simulink model "slexHARFixedPointExample"  (R2023a)
settings: Solver=FixedStepAuto  StartTime=0.0  StopTime=numSteps  FixedStep=1  RelTol=1e-3
PreLoadFcn:
  | % Pre-processing parameters
  | s = [1.0000   -1.0000         0    1.0000   -0.9004         0
  |     1.0000   -1.9996    1.0000    1.0000   -1.9203    0.9254
  |     1.0000   -1.9990    1.0000    1.0000   -1.9762    0.9791
  |     1.0000   -1.9986    1.0000    1.0000   -1.9929    0.9953];
  | 
  | fs = 10;
  | g = 0.9013;
  | featsDT = single(1);
  | lags = (0:32)';
  | tc = (1/fs)*lags;
undefined symbols (not defined in the file or in its folder): dfilt
libraries: dspstat3 x3, statsLibrary x1, dsparch4 x1, dspsigops x1
settings Model: Creator=The MathWorks, Inc.  LastModifiedBy=The MathWorks, Inc.
settings SolverCC: AlgebraicLoopSolver=TrustRegion
settings DataIOCC: ExternalInput=ts  LoadExternalInput=on
settings OptimizationCC: DefaultParameterBehavior=Inlined  EnhancedBackFolding=on  PassReuseOutputArgsAs=Individual arguments  ZeroExternalMemoryAtStartup=off  ZeroInternalMemoryAtStartup=off  OptimizeBlockOrder=speed  DifferentSizesBufferReuse=on  OptimizationCustomize=off  EfficientTunableParamExpr=on
settings DebuggingCC: SignalRangeChecking=warning  ParameterTunabilityLossMsg=error  UnconnectedInputMsg=warning  UnconnectedOutputMsg=warning  UnconnectedLineMsg=warning
settings ModelReferenceCC: EnableRefExpFcnMdlSchedulingChecks=on
settings SFSimCC: MATLABDynamicMemAlloc=off
settings RTWCC: Description=Embedded Coder  SystemTargetFile=ert.tlc  GenCodeOnly=on  TemplateMakefile=ert_default_tmf  GenerateCodeMetricsReport=on  DLArmComputeVersion=19.05
settings CodeAppCC: ForceParamTrailComments=on  IgnoreCustomStorageClasses=off  OperatorAnnotations=on  SimulinkDataObjDesc=on  SFDataObjDesc=on  InsertBlockDesc=on
settings ERTTargetCC: TargetLangStandard=C99 (ISO)  GenerateSampleERTMain=on  SupportComplex=off  SupportVariableSizeSignals=on  InlinedParameterPlacement=NonHierarchical  ERTCustomFileTemplate=example_file_process.tlc

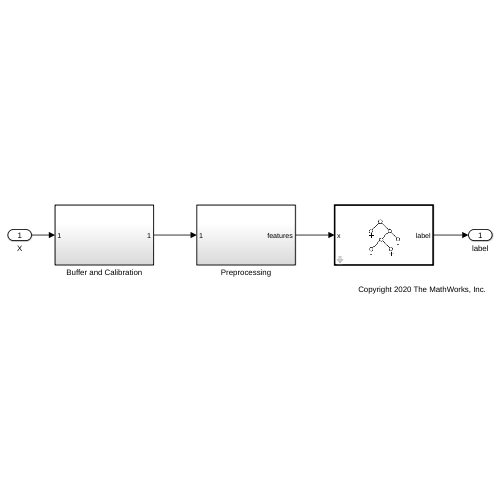
[thumbnail: Simulink's stored preview of the top-level diagram]
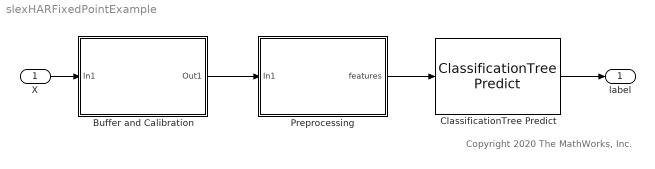
== system slexHARFixedPointExample ==
  note: Copyright 2020 The MathWorks, Inc.
  X : Inport  OutDataTypeStr=double  PortDimensions=[1,3]  SampleTime=1
  Buffer and Calibration : Subsystem
  ClassificationTree Predict : statsLibrary/Classification/ClassificationTree Predict  TrainedLearner=classificationTree  ShowOutputScore=off  LabelDataTypeStr=Inherit: Inherit via back propagation  LabelOutMin=[]  LabelOutMax=[]  ScoreOutMin=[]  ScoreOutMax=[]  RawScoreOutMin=[]  RawScoreOutMax=[]  StoredEnumName=treeMdl_enumLabels
  Preprocessing : Subsystem
  label : Outport
  wires:
  Preprocessing/1(features) -> ClassificationTree Predict/1
  ClassificationTree Predict/1 -> label/1
  X/1 -> Buffer and Calibration/1(In1)
  Buffer and Calibration/1(Out1) -> Preprocessing/1(In1)

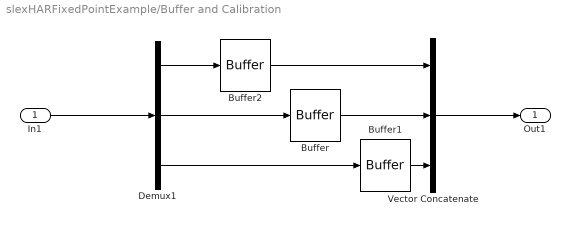
== system slexHARFixedPointExample/Buffer and Calibration ==
  In1 : Inport
  Buffer : Buffer  N=32  V=12  OutputFrames=off
  Buffer1 : Buffer  N=32  V=12  OutputFrames=off
  Buffer2 : Buffer  N=32  V=12  OutputFrames=off
  Demux1 : Demux  Outputs=3
  Vector Concatenate : Concatenate  NumInputs=3  Mode=Multidimensional array  ConcatenateDimension=2
  Out1 : Outport
  wires:
  Buffer1/1 -> Vector Concatenate/3
  Buffer2/1 -> Vector Concatenate/1
  In1/1 -> Demux1/1
  Demux1/3 -> Buffer1/1
  Buffer/1 -> Vector Concatenate/2
  Vector Concatenate/1 -> Out1/1
  Demux1/1 -> Buffer2/1
  Demux1/2 -> Buffer/1

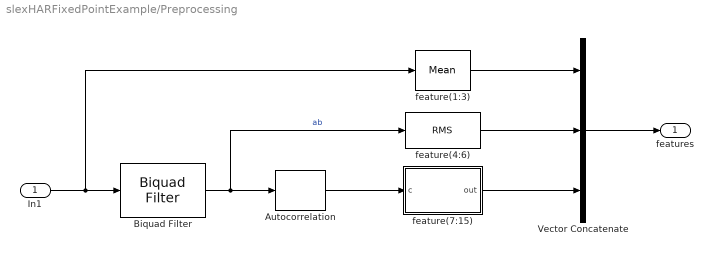
== system slexHARFixedPointExample/Preprocessing ==
  In1 : Inport
  Autocorrelation : dspstat3/Autocorrelation  AllPositiveLags=on  maxlag=1  bias=None  domain=Time  roundingMode=Floor  overflowMode=off  outputDataTypeStr=Inherit: Same as accumulator  outputMin=[]  outputMax=[]  outputLastDataTypeStr=Inherit: Same as accumulator
  Biquad Filter : dsparch4/Biquad Filter  FilterSource=Dialog parameters  CoeffSource=Specify via dialog  FilterObject=dfilt.df2tsos([1 0.3 0.4],[1 0.1 0.2])  IIRFiltStruct=Direct form II transposed  BiQuadCoeffs=s  ScaleValues=g  IC=0  ICnum=0  ICden=0  a0Flag=Warning  optimizeScaleValues=on  ScaleValueMode=Specify via input port (g)  roundingMode=Floor  overflowMode=off  scaleValueFracLength=14  denProdOutputFracLength=30  denAccumFracLength=30  secondMemoryFracLength=15
  Vector Concatenate : Concatenate  NumInputs=3
  feature(1:3) : dspstat3/Mean  run=off  InputProcessing=Columns as channels (frame based)  reset_popup=None  directionMode=Each column  dimension=1  roiEnable=off  roiType=Rectangles  roiPortion=Entire ROI  roiOutput=Individual statistics for each ROI  roiFlag=off  roundingMode=Floor  overflowMode=off  outputDataTypeStr=Inherit: Same as accumulator  outputMin=[]  outputMax=[]  outputLastDataTypeStr=Inherit: Same as accumulator
  feature(4:6) : dspstat3/RMS  run=off  directionMode=Each column  dimension=1  InputProcessing=Columns as channels (frame based)  reset_popup=None
  feature(7:15) : Subsystem
  features : Outport
  wires:
  In1/1 -> feature(1:3)/1, Biquad Filter/1
  Biquad Filter/1 -> feature(4:6)/1, Autocorrelation/1  "ab"
  Autocorrelation/1 -> feature(7:15)/1(c)
  feature(1:3)/1 -> Vector Concatenate/1
  feature(4:6)/1 -> Vector Concatenate/2
  feature(7:15)/1(out) -> Vector Concatenate/3
  Vector Concatenate/1 -> features/1

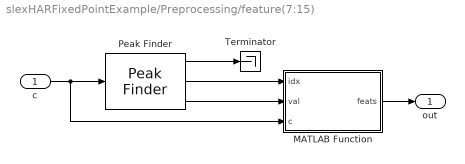
== system slexHARFixedPointExample/Preprocessing/feature(7:15) ==
  c : Inport
  MATLAB Function : MATLAB Function  TreatAsAtomicUnit=on
  Peak Finder : dspsigops/Peak Finder  polarity=Maxima  indexBase=One  outputIdx=on  outputVal=on  maxPeaks=10  NoiseDistinguish=on  thresh=0.0005  roundingMode=Floor  overflowMode=off
      settings: allowOverrides=off
  Terminator : Terminator
  out : Outport
  wires:
  c/1 -> MATLAB Function/3(c), Peak Finder/1
  Peak Finder/1 -> Terminator/1
  Peak Finder/2 -> MATLAB Function/1(idx)
  Peak Finder/3 -> MATLAB Function/2(val)
  MATLAB Function/1(feats) -> out/1

== matlab function slexHARFixedPointExample/Preprocessing/feature(7:15)/MATLAB Function ==
  data: idx input; val input; c input; feats output; tc parameter
function feats = fcn(idx,val,c,tc)
feats = zeros(9,1,'like',val);
for k = 1:3
%     [pks,locs] = findpeaks([0;c(:,k)],...
%         'minpeakprominence',minprom,...
%         'minpeakdistance',minpkdist);
    nzInds = idx(:,k)>0;
    locs = idx(nzInds,k);
    pks = val(nzInds,k);
    
    tcl = tc(locs);

    % Feature 1 - peak height at 0
    feats(3*(k-1)+1) = c(1,k);
    % Features 2 and 3 - position and height of first peak 
    if(length(tcl) >= 2)   % else f2,f3 already 0
        feats(3*(k-1)+2) = tcl(2);
        feats(3*(k-1)+3) = pks(2);
    end
end
